simulink model "SlidingModeControl"  (R2020a)
settings: Solver=VariableStepAuto  StartTime=0.0  StopTime=10.0  RelTol=1e-3
libraries: simulink x1
settings Model: Creator=shita  LastModifiedBy=shita

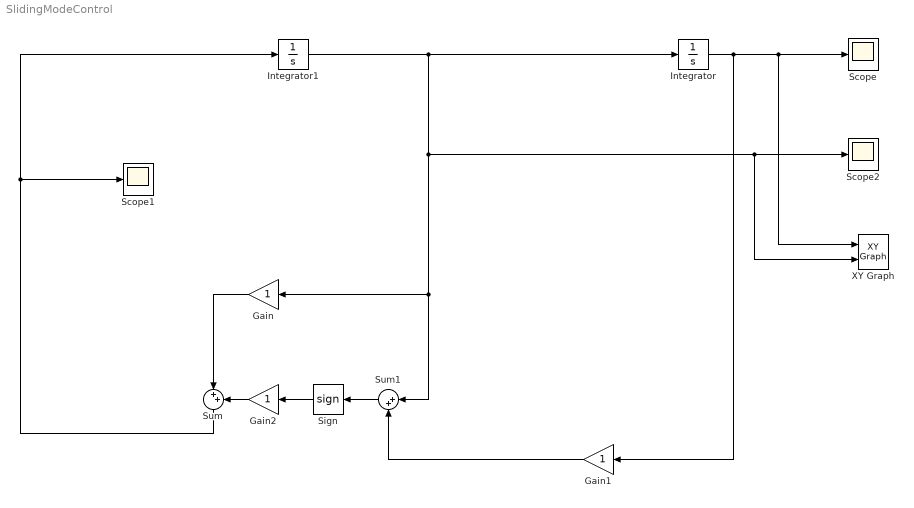
== system SlidingModeControl ==
  Gain : Gain
  Gain1 : Gain
  Gain2 : Gain
  Integrator : Integrator
  Integrator1 : Integrator
  Scope : Scope
  Scope1 : Scope
  Scope2 : Scope
  Sign : Signum
  Sum : Sum  Inputs=|++
  Sum1 : Sum  Inputs=|++
  XY Graph : simulink/Sinks/XY Graph  xmin=-1  xmax=1  ymin=-1  ymax=1  st=-1
  wires:
  Integrator1/1 -> Integrator/1, XY Graph/2, Scope2/1, Sum1/1, Gain/1
  Integrator/1 -> XY Graph/1, Scope/1, Gain1/1
  Gain/1 -> Sum/1
  Gain1/1 -> Sum1/2
  Sum/1 -> Scope1/1, Integrator1/1
  Gain2/1 -> Sum/2
  Sum1/1 -> Sign/1
  Sign/1 -> Gain2/1
